simulink model "IEEE13_dstatcom"  (R2024b)
settings: Solver=ode4  StartTime=0.0  StopTime=1.3  FixedStep=Ts  MaxStep=1e-4  RelTol=1e-4
InitFcn:
  | a=1; % Loading Factor
  | Ts=50e-6;
  | % phase to sequence conversion of RXB matrices
  | c=1*exp(sqrt(-1)*(120*pi/180));
  | T=[1 1 1;1 c*c c;1 c c*c];
  | Tinv=1/3*[1 1 1;1 c c*c;1 c*c c];
  | 
  | % Simulation data for the IEEE 13 Node Test Feeder model
  | mi2km = 1.60934;%  miles to km conversion
  | ft2km = 0.0003048; % feet to km conversion
  | ms2F = 1*1e-6/(2*pi*60);% microsiemens to Farads conversion
  | 
  | 
  | %% Configuration 601
  | % Series Resitance and Reactance - ohm/mile
  | R_601 = [0.3465 0.1560 0.1580;0.1560 0.3375 0.1535;0.1580 0.1535 0.3414];
  | X_601 = [1.1079 0.5017 0.4236;0.5017 1.0478 0.3849;0.4236 0.3849 1.0348];
  | % charging susceptance - microsiemens/mile
  | B_601 = [6.2998 -1.9958 -1.2595;-1.9958 5.9597 -0.7417;-1.2595 -0.7417 5.6386];
  | 
  | R_601 = R_601/mi2km;
  | Rseq=Tinv*R_601*T;
  | R1_601=Rseq(2,2);R0_601=Rseq(1,1);
  | 
  | L_601 = (X_601/(2*pi*60))/mi2km;
  | Lseq=Tinv*L_601*T;
  | L1_601=Lseq(2,2);L0_601=Lseq(1,1);
  | 
  | C_601 =(B_601*ms2F)/mi2km;
  | Cseq=Tinv*C_601*T;
  | C1_601=Cseq(2,2);C0_601=Cseq(1,1);
  | 
  | %% Configuration 602 - series reactance - ohm/mile
  | R_602 = [0.7526 0.1580 0.1560;0.1580 0.7475 0.1535;0.1560 0.1535 0.7436];
  | X_602 = [1.1814 0.4236 0.5017;0.4236 1.1983 0.3849;0.5017 0.3849 1.2112];
  | % charging susceptance - microsiemens/mile
  | B_602 = [5.6990 -1.0817 -1.6905;-1.0817 5.1795 -0.6588;-1.6905 -0.6588 5.4246];
  | 
  | R_602 = R_602/mi2km;
  | Rseq=Tinv*R_602*T;
  | R1_602=Rseq(2,2);R0_602=Rseq(1,1);
  | 
  | L_602 = (X_602/(2*pi*60))/mi2km;
  | Lseq=Tinv*L_602*T;
  | L1_602=Lseq(2,2);L0_602=Lseq(1,1);
  | 
  | C_602 =(B_602*ms2F)/mi2km;
  | Cseq=Tinv*C_602*T;
  | C1_602=Cseq(2,2);C0_602=Cseq(1,1);
  | %% Configuration 603 - series reactance - ohm/mile
  | R_603 = [0 0 0;0 1.3294 0.2066;0 0.2066 1.3238];
  | X_603 = [0 0 0;0 1.3471 0.4591;0 0.4591 1.3569];
  | % charging susceptance - microsiemens/mile
  | B_603 = [0 0 0;0 4.7097 -0.8999;0 -0.8999 4.6658];
  | 
  | % convert for SPS
  | R_603 = R_603/mi2km;
  | Rseq=Tinv*R_603*T;
  | R1_603=Rseq(2,2);R0_603=Rseq(1,1);
  | 
  | ... (+71 lines)
undefined symbols (not defined in the file): find_system
libraries: spsGroundLib x46, spsSeriesRLCBranchLib x44, spsThreePhaseVIMeasurementLib x17, spsThreePhaseSeriesRLCLoadLib x7, spsControlledVoltageSourceLib x6, spsVoltageMeasurementLib x6, spsOnDelayLib x6, spsThreePhasePISectionLineLib x5, spsSeriesRLCLoadLib x5, spsMutualInductanceLib x4, spsRMSLib x4, spsThreePhaseBreakerLib x3
(part 3 of 3)

== system IEEE13_dstatcom/Regulator 1/Single Phase SVR_C/Voltage Regulator Control/Tap Changer Control/Edge Detector ==
  note: Edge or Slope Detector
  In : Inport
  Constant1 : Constant  Value=model
  Demux : Demux  Outputs=2
      settings: DisplayOption=none
  Logical Operator1 : Logic  Operator=OR
  Memory : Memory  InitialCondition=ic  LinearizeAsDelay=on
  Multiport Switch : MultiPortSwitch  InputSameDT=off
  NEGATIVE Edge : Subsystem  TreatAsAtomicUnit=on
  POSITIVE Edge : Subsystem  TreatAsAtomicUnit=on
  either edge : Constant  Value=[1 1]
  neg. edge : Constant  Value=[0 1]
  pos. edge : Constant  Value=[1 0]
  Out : Outport  VectorParamsAs1DForOutWhenUnconnected=off
  wires:
  Logical Operator1/1 -> Out/1
  NEGATIVE Edge/1(OUT) -> Logical Operator1/2
  POSITIVE Edge/1(OUT) -> Logical Operator1/1
  Memory/1 -> POSITIVE Edge/2(IN previous), NEGATIVE Edge/2(IN previous)
  In/1 -> POSITIVE Edge/1(IN), NEGATIVE Edge/1(IN), Memory/1
  pos. edge/1 -> Multiport Switch/2
  neg. edge/1 -> Multiport Switch/3
  Constant1/1 -> Multiport Switch/1
  Multiport Switch/1 -> Demux/1
  Demux/1 -> POSITIVE Edge/Enable
  Demux/2 -> NEGATIVE Edge/Enable
  either edge/1 -> Multiport Switch/4

== system IEEE13_dstatcom/Regulator 1/Single Phase SVR_A/Voltage Regulator Control/Tap Changer Control/Edge Detector/NEGATIVE Edge ==
  IN : Inport
  IN previous : Inport  Port=2
  Enable : EnablePort  PropagateVarSize=During execution
  Relational Operator1 : RelationalOperator  Operator=>
  OUT : Outport  VectorParamsAs1DForOutWhenUnconnected=off
  wires:
  Relational Operator1/1 -> OUT/1
  IN previous/1 -> Relational Operator1/1
  IN/1 -> Relational Operator1/2

== system IEEE13_dstatcom/Regulator 1/Single Phase SVR_A/Voltage Regulator Control/Tap Changer Control/Edge Detector/POSITIVE Edge ==
  IN : Inport
  IN previous : Inport  Port=2
  Enable : EnablePort  PropagateVarSize=During execution
  Relational Operator1 : RelationalOperator  Operator=>
  OUT : Outport  VectorParamsAs1DForOutWhenUnconnected=off
  wires:
  Relational Operator1/1 -> OUT/1
  IN previous/1 -> Relational Operator1/2
  IN/1 -> Relational Operator1/1

== system IEEE13_dstatcom/Regulator 1/Single Phase SVR_B/Voltage Regulator Control/Tap Changer Control/Edge Detector/NEGATIVE Edge ==
  IN : Inport
  IN previous : Inport  Port=2
  Enable : EnablePort  PropagateVarSize=During execution
  Relational Operator1 : RelationalOperator  Operator=>
  OUT : Outport  VectorParamsAs1DForOutWhenUnconnected=off
  wires:
  IN/1 -> Relational Operator1/2
  IN previous/1 -> Relational Operator1/1
  Relational Operator1/1 -> OUT/1

== system IEEE13_dstatcom/Regulator 1/Single Phase SVR_B/Voltage Regulator Control/Tap Changer Control/Edge Detector/POSITIVE Edge ==
  IN : Inport
  IN previous : Inport  Port=2
  Enable : EnablePort  PropagateVarSize=During execution
  Relational Operator1 : RelationalOperator  Operator=>
  OUT : Outport  VectorParamsAs1DForOutWhenUnconnected=off
  wires:
  IN/1 -> Relational Operator1/1
  IN previous/1 -> Relational Operator1/2
  Relational Operator1/1 -> OUT/1

== system IEEE13_dstatcom/Regulator 1/Single Phase SVR_C/Voltage Regulator Control/Tap Changer Control/Edge Detector/NEGATIVE Edge ==
  IN : Inport
  IN previous : Inport  Port=2
  Enable : EnablePort  PropagateVarSize=During execution
  Relational Operator1 : RelationalOperator  Operator=>
  OUT : Outport  VectorParamsAs1DForOutWhenUnconnected=off
  wires:
  Relational Operator1/1 -> OUT/1
  IN previous/1 -> Relational Operator1/1
  IN/1 -> Relational Operator1/2

== system IEEE13_dstatcom/Regulator 1/Single Phase SVR_C/Voltage Regulator Control/Tap Changer Control/Edge Detector/POSITIVE Edge ==
  IN : Inport
  IN previous : Inport  Port=2
  Enable : EnablePort  PropagateVarSize=During execution
  Relational Operator1 : RelationalOperator  Operator=>
  OUT : Outport  VectorParamsAs1DForOutWhenUnconnected=off
  wires:
  Relational Operator1/1 -> OUT/1
  IN previous/1 -> Relational Operator1/2
  IN/1 -> Relational Operator1/1

== matlab function IEEE13_dstatcom/D-STATCOM/DST Controller ==
  settings: updateMethod=DISCRETE  sampleTime=50e-6
  data: vpcc input; vinv output; iL input; ic input; en input; mode input; g input; dbg output
function [vinv, dbg] = dstatcom_controller(vpcc, iL, ic, en, mode, g)
% D-STATCOM control in the synchronous reference frame with PI regulators.
% The text of this file is copied into the MATLAB Function block of
% IEEE13_dstatcom.slx by build_dstatcom.
%
%   vpcc  phase-to-ground voltage at the point of connection (V)
%   iL    load current (A)
%   ic    D-STATCOM current, positive into the point of connection (A)
%   en    1 = controller active, 0 = track the grid voltage (no current)
%   mode  1 = cancel load reactive power, harmonics and unbalance
%         2 = regulate the voltage magnitude, plus harmonics and unbalance
%   g     gains: [current-loop bandwidth (Hz); KpDc; KiDc; KpV; KiV]
%         hand-tuned baseline: [1500; 1; 15; 5; 500]
%
%   vinv  inverter voltage command for the averaged converter (V)
%   dbg   [Vdc; idRef; iqRef; id; iq; Vd; theta; f]
%
% The converter is an averaged model: no switching, and the DC link is
% represented by its power balance, C*Vdc*dVdc/dt = -Pac.
%#codegen

Ts = 50e-6; w0 = 2*pi*60;
L = 0.2e-3; R = 5e-3; C = 10e-3;          % coupling filter and DC capacitor
VdcRef = 1000;                            % V
Imax = 850;                               % A peak, about 500 kVA at 480 V
Vref = 480*sqrt(2/3);                     % V peak, 1 pu phase voltage
N = 333;                                  % samples in one fundamental cycle

KpI = 2*pi*g(1)*L;  KiI = 2*pi*g(1)*R;    % current loops
KpDc = g(2);        KiDc = g(3);          % DC-link voltage loop, A/V
KpV = g(4);         KiV = g(5);           % AC voltage loop, A/V
KpPll = 178;        KiPll = 15791;        % PLL, 20 Hz bandwidth

persistent theta xPll xId xIq xDc xV vdc buf bsum idx
if isempty(theta)
    theta = atan2((vpcc(2) - vpcc(3))/sqrt(3), (2*vpcc(1) - vpcc(2) - vpcc(3))/3);
    xPll = 0; xId = 0; xIq = 0; xDc = 0; xV = 0; vdc = VdcRef;
    buf = zeros(N, 4); buf(:, 4) = VdcRef;
    bsum = [0; 0; 0; N*VdcRef];
    idx = 1;
end

% Phase-locked loop on the connection-point voltage
[vd, vq] = abc2dq(vpcc, theta);
vmag = max(hypot(vd, vq), 1);
ePll = vq / vmag;
w = w0 + KpPll*ePll + xPll;

[iLd, iLq] = abc2dq(iL, theta);
[icd, icq] = abc2dq(ic, theta);

% One-cycle moving averages: fundamental active and reactive load current,
% voltage magnitude and DC-link voltage
s = [iLd; iLq; vd; vdc];
bsum = bsum + s - buf(idx, :)';
buf(idx, :) = s';
idx = mod(idx, N) + 1;
avg = bsum / N;

if en < 0.5
    vinv = vpcc;
    xId = 0; xIq = 0; xDc = 0; xV = 0;
    idRef = 0; iqRef = 0;
else
    % DC-link voltage PI: active current drawn from the grid
    eDc = VdcRef - avg(4);
    idc = sat(KpDc*eDc + xDc, 0.3*Imax);
    xDc = sat(xDc + KiDc*eDc*Ts, 0.3*Imax);

    idRef = (iLd - avg(1)) - idc;
    if mode < 1.5
        iqRef = iLq;
    else
        % AC voltage PI: negative q current injects reactive power
        eV = Vref - avg(3);
        iqv = sat(KpV*eV + xV, Imax);
        xV = sat(xV + KiV*eV*Ts, Imax);
        iqRef = (iLq - avg(2)) - iqv;
    end
    m = hypot(idRef, iqRef);
    if m > Imax
        idRef = idRef*Imax/m; iqRef = iqRef*Imax/m;
    end

    % Current PI loops with voltage feed-forward and cross-coupling terms
    eD = idRef - icd; eQ = iqRef - icq;
    vdCmd = vd + KpI*eD + xId - w*L*icq;
    vqCmd = vq + KpI*eQ + xIq + w*L*icd;
    vlim = vdc / sqrt(3);
    vm = hypot(vdCmd, vqCmd);
    if vm > vlim
        vdCmd = vdCmd*vlim/vm; vqCmd = vqCmd*vlim/vm;
    else
        xId = xId + KiI*eD*Ts; xIq = xIq + KiI*eQ*Ts;
    end

    % The output reaches the network one sample later: advance the angle
    vinv = dq2abc(vdCmd, vqCmd, theta + 1.5*w*Ts);

    pac = 1.5*(vdCmd*icd + vqCmd*icq);
    vdc = max(vdc - Ts*pac/(C*vdc), 100);
end

dbg = [vdc; idRef; iqRef; icd; icq; vd; theta; w/(2*pi)];

xPll = xPll + KiPll*ePll*Ts;
theta = mod(theta + w*Ts, 2*pi);
end

function [d, q] = abc2dq(x, th)
al = (2*x(1) - x(2) - x(3)) / 3;
be = (x(2) - x(3)) / sqrt(3);
d =  al*cos(th) + be*sin(th);
q = -al*sin(th) + be*cos(th);
end

function x = dq2abc(d, q, th)
al = d*cos(th) - q*sin(th);
be = d*sin(th) + q*cos(th);
x = [al; -al/2 + sqrt(3)/2*be; -al/2 - sqrt(3)/2*be];
end

function y = sat(u, lim)
y = min(max(u, -lim), lim);
end
